simulink model "kalmanFilter"  (R2023b)
settings: Solver=VariableStepAuto  StartTime=0.0  StopTime=10.0  RelTol=1e-3
undefined symbols (not defined in the file or in its folder): dt_KF, P0, Q
libraries: rotationConversionLib x1, matrix_library x1
settings Model: Creator=kristopherriordan  LastModifiedBy=kristopherriordan

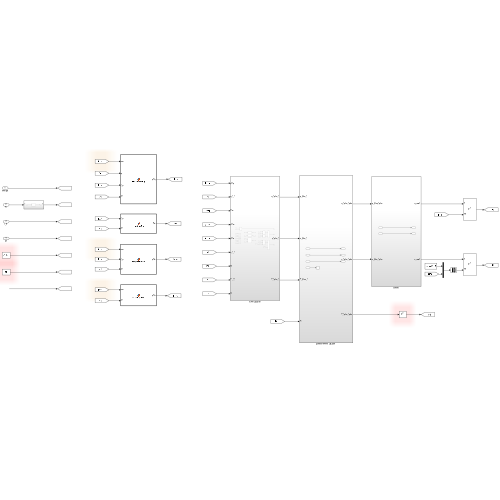
[thumbnail: Simulink's stored preview of the top-level diagram]
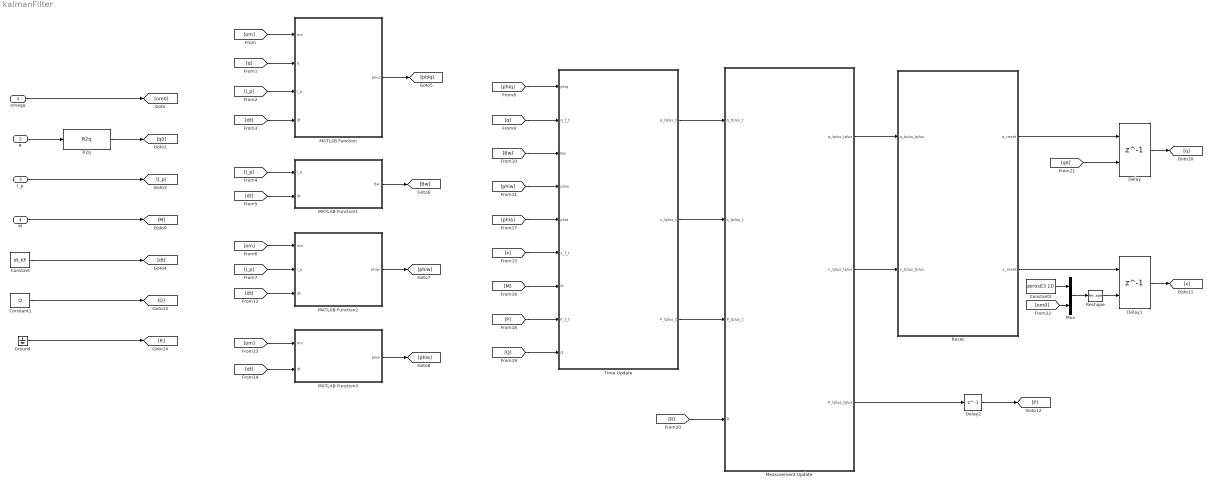
== system kalmanFilter ==
  omega : Inport
  R : Inport  Port=2
  I_p : Inport  Port=3
  M : Inport  Port=4
  Constant : Constant  Value=dt_KF
  Constant1 : Constant  Value=Q
  Constant2 : Constant  Value=zeros([3 1])
  Delay : Delay  DelayLength=1  InitialConditionSource=Input port  InitialCondition=0
      settings: InputPortMap=u0,p4
  Delay1 : Delay  DelayLength=1  InitialConditionSource=Input port  InitialCondition=0
      settings: InputPortMap=u0,p4
  Delay2 : Delay  DelayLength=1  InitialCondition=P0
  Ground : Ground
  MATLAB Function : MATLAB Function  TreatAsAtomicUnit=on
  MATLAB Function1 : MATLAB Function  TreatAsAtomicUnit=on
  MATLAB Function2 : MATLAB Function  TreatAsAtomicUnit=on
  MATLAB Function3 : MATLAB Function  TreatAsAtomicUnit=on
  "Measurement Update " : Subsystem
  Mux : Mux  Inputs=2
  R2q : rotationConversionLib/R2q  SystemSampleTime=-1  VariantActivationTime=update diagram  AllowFlexibleInterface=on  Latency=0  AutoFrameSizeCalculation=off
  Reset : Subsystem
  Reshape : Reshape  OutputDimensionality=Column vector (2-D)
  Time Update : Subsystem
  wires:
  R/1 -> R2q/1
  omega/1 -> [om0]
  R2q/1 -> [q0]
  Constant/1 -> [dt]
  I_p/1 -> [I_p]
  [om] -> MATLAB Function/1(om)
  [q] -> MATLAB Function/2(q)
  [I_p] -> MATLAB Function/3(I_p)
  [dt] -> MATLAB Function/4(dt)
  [I_p] -> MATLAB Function1/1(I_p)
  [dt] -> MATLAB Function1/2(dt)
  MATLAB Function/1(phiq) -> [phiq]
  MATLAB Function1/1(Bw) -> [Bw]
  [om] -> MATLAB Function2/1(om)
  [I_p] -> MATLAB Function2/2(I_p)
  MATLAB Function2/1(phiw) -> [phiw]
  [phiq] -> Time Update/1(phiq)
  [q] -> Time Update/2(q_t_t)
  [Bw] -> Time Update/3(Bw)
  [phiw] -> Time Update/4(phiw)
  [dt] -> MATLAB Function2/3(dt)
  [om] -> MATLAB Function3/1(om)
  [dt] -> MATLAB Function3/2(dt)
  MATLAB Function3/1(phia) -> [phia]
  [x] -> Time Update/6(x_t_t)
  M/1 -> [M]
  [M] -> Time Update/7(M)
  Time Update/1(q_tplus_t) -> "Measurement Update "/1(q_tplus_t)
  Time Update/2(x_tplus_t) -> "Measurement Update "/2(x_tplus_t)
  "Measurement Update "/1(q_tplus_tplus) -> Reset/1(q_tplus_tplus)
  "Measurement Update "/2(x_tplus_tplus) -> Reset/2(x_tplus_tplus)
  Reset/1(q_reset) -> Delay/1
  Reset/2(x_reset) -> Delay1/1
  Delay/1 -> [q]
  [phia] -> Time Update/5(phia)
  Time Update/3(P_tplus_t) -> "Measurement Update "/3(P_tplus_t)
  Delay1/1 -> [x]
  "Measurement Update "/3(P_tplus_tplus) -> Delay2/1
  Delay2/1 -> [P]
  [P] -> Time Update/8(P_t_t)
  Constant1/1 -> [Q]
  [Q] -> Time Update/9(Q)
  Ground/1 -> [R]
  [R] -> "Measurement Update "/4(R)
  [q0] -> Delay/2
  Reshape/1 -> Delay1/2
  Mux/1 -> Reshape/1
  [om0] -> Mux/2
  Constant2/1 -> Mux/1

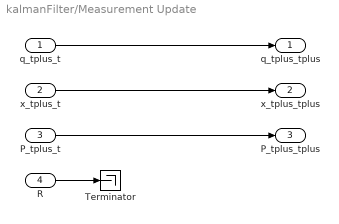
== system kalmanFilter/Measurement Update  ==
  q_tplus_t : Inport
  x_tplus_t : Inport  Port=2
  P_tplus_t : Inport  Port=3
  R : Inport  Port=4
  Terminator : Terminator
  q_tplus_tplus : Outport
  x_tplus_tplus : Outport  Port=2
  P_tplus_tplus : Outport  Port=3
  wires:
  q_tplus_t/1 -> q_tplus_tplus/1
  x_tplus_t/1 -> x_tplus_tplus/1
  P_tplus_t/1 -> P_tplus_tplus/1
  R/1 -> Terminator/1

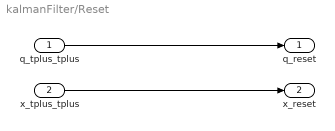
== system kalmanFilter/Reset ==
  q_tplus_tplus : Inport
  x_tplus_tplus : Inport  Port=2
  q_reset : Outport
  x_reset : Outport  Port=2
  wires:
  q_tplus_tplus/1 -> q_reset/1
  x_tplus_tplus/1 -> x_reset/1

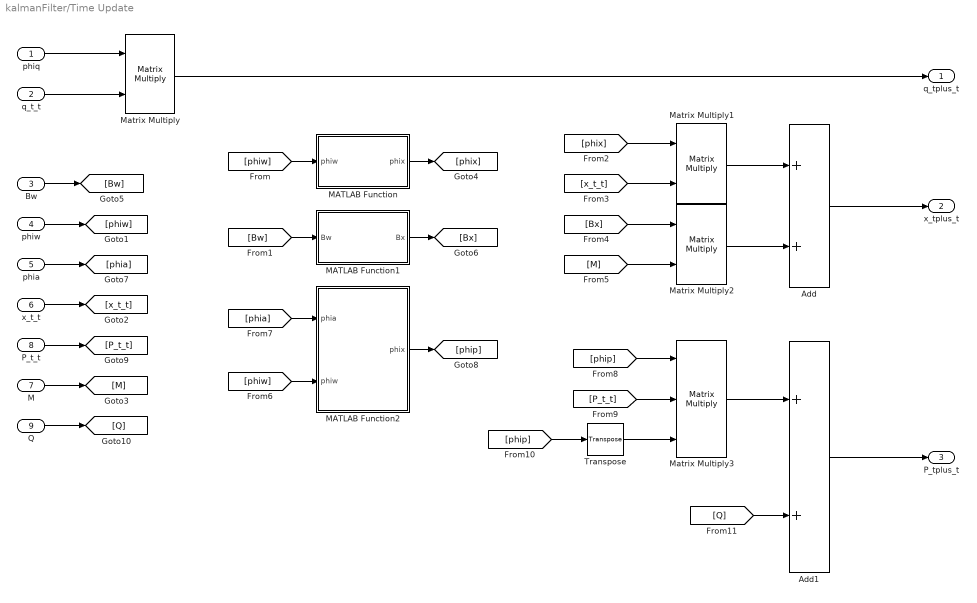
== system kalmanFilter/Time Update ==
  phiq : Inport
  q_t_t : Inport  Port=2
  Bw : Inport  Port=3
  phiw : Inport  Port=4
  phia : Inport  Port=5
  x_t_t : Inport  Port=6
  M : Inport  Port=7
  P_t_t : Inport  Port=8
  Q : Inport  Port=9
  Add : Sum
  Add1 : Sum
  MATLAB Function : MATLAB Function  TreatAsAtomicUnit=on
  MATLAB Function1 : MATLAB Function  TreatAsAtomicUnit=on
  MATLAB Function2 : MATLAB Function  TreatAsAtomicUnit=on
  Matrix Multiply : Product  Multiplication=Matrix(*)
  Matrix Multiply1 : Product  Multiplication=Matrix(*)
  Matrix Multiply2 : Product  Multiplication=Matrix(*)
  Matrix Multiply3 : Product  Inputs=***  Multiplication=Matrix(*)
  Transpose : matrix_library/Transpose
  q_tplus_t : Outport
  x_tplus_t : Outport  Port=2
  P_tplus_t : Outport  Port=3
  wires:
  phiq/1 -> Matrix Multiply/1
  q_t_t/1 -> Matrix Multiply/2
  Matrix Multiply/1 -> q_tplus_t/1
  Bw/1 -> [Bw]
  phiw/1 -> [phiw]
  x_t_t/1 -> [x_t_t]
  M/1 -> [M]
  [phiw] -> MATLAB Function/1(phiw)
  [Bw] -> MATLAB Function1/1(Bw)
  MATLAB Function/1(phix) -> [phix]
  MATLAB Function1/1(Bx) -> [Bx]
  [phix] -> Matrix Multiply1/1
  [x_t_t] -> Matrix Multiply1/2
  [Bx] -> Matrix Multiply2/1
  [M] -> Matrix Multiply2/2
  Matrix Multiply1/1 -> Add/1
  Matrix Multiply2/1 -> Add/2
  Add/1 -> x_tplus_t/1
  phia/1 -> [phia]
  [phiw] -> MATLAB Function2/2(phiw)
  [phia] -> MATLAB Function2/1(phia)
  MATLAB Function2/1(phix) -> [phip]
  P_t_t/1 -> [P_t_t]
  [phip] -> Matrix Multiply3/1
  [P_t_t] -> Matrix Multiply3/2
  Transpose/1 -> Matrix Multiply3/3
  [phip] -> Transpose/1
  Matrix Multiply3/1 -> Add1/1
  Q/1 -> [Q]
  [Q] -> Add1/2
  Add1/1 -> P_tplus_t/1

== matlab function kalmanFilter/MATLAB Function1 ==
  data: I_p input; Bw output; dt input
function Bw = constructBw(I_p, dt)

Ixyz = diat(I_p);
Ix = Ixyz(1);
Iy = Ixyz(2);
Iz = Ixyz(3);

Bw = dt.*[1/Ix, 0, 0;
          0, 1/Iy, 0;
          0, 0, 1/Iz];

% B = [Bw;zeros([4 3])];

== matlab function kalmanFilter/MATLAB Function ==
  data: om input; phiq output; q input; I_p input; dt input
function phiq = constructPhiQ(om, q, I_p, dt)

om1 = om(1);
om2 = om(2);
om3 = om(3);
ommag = norm(om);

q0 = q(1);
q1 = q(2);
q2 = q(3);
q3 = q(4);

Ixyz = diag(I_p);
Ix = Ixyz(1);
Iy = Ixyz(2);
Iz = Ixyz(3);

C = cos(ommag*dt/2);
S = (1/(ommag + 1e-10))*sin(ommag*dt/2);

% phiw = [1, (Iy - Iz)*om3/Ix, (Iy-Iz)*om2/Ix;
        (Iz - Ix)*om3/Iy, 1, (Iz - Ix)*om1/Iy;
        (Ix - Iy)*om2/Iz, (Ix - Iy)*om1/Iz, 1];

phiq = [-S*q1, -S*q2, -S*q3, C, -S*om1, -S*om2, -S*wom3;
        S*q0, -S*q3, S*q2, S*om1, C, S*om3, -S*om2;
        S*q3, S*q0, -S*q1, S*om2, -S*om3, C, S*om1;
        -S*q2, S*q1, S*q0, S*om3, S*om2, -S*om1, C];

% phi = [phiw, zeros([3 4]);phiq];

== matlab function kalmanFilter/MATLAB Function2 ==
  data: om input; phiw output; I_p input; dt input
function phiw = consructPhiOm(om, I_p, dt)

Ixyz = diag(I_p);
Ix = Ixyz(1);
Iy = Ixyz(2);
Iz = Ixyz(3);

om1 = om(1);
om2 = om(2);
om3 = om(3);


phiw = dt.*[1, (Iy - Iz)*om3/Ix, (Iy-Iz)*om2/Ix;
        (Iz - Ix)*om3/Iy, 1, (Iz - Ix)*om1/Iy;
        (Ix - Iy)*om2/Iz, (Ix - Iy)*om1/Iz, 1];

== matlab function kalmanFilter/MATLAB Function3 ==
  data: om input; phia output; dt input
function phia = constructPhiA(om, dt)

om1 = om(1);
om2 = om(2);
om3 = om(3);

omcross = [0 -om3 om2;
           om3 0 -om1;
           -om2 om1 0];

ommag = norm(om);

C = cos(ommag*dt/2);
S = (1/(ommag + 1e-10))*sin(ommag*dt/2);

phia = eye(3) + S.*omcross + ((1 - C)/ommag^2).*omcross*omcross;

== matlab function kalmanFilter/Time Update/MATLAB Function ==
  data: phiw input; phix output
function phix = constructPhiX(phiw)

phix = [eye(3), zeros([3 3]);
        zeros([3 3]), phiw];

== matlab function kalmanFilter/Time Update/MATLAB Function1 ==
  data: Bw input; Bx output
function Bx = constructBx(Bw)

Bx = [zeros([3 3]);
      Bw];

== matlab function kalmanFilter/Time Update/MATLAB Function2 ==
  data: phia input; phiw input; phix output
function phix = constructPhiX(phia, phiw)

phix = [phia, zeros([3 3]);
        zeros([3 3]), phiw];
